simulink model "HW6SimulinkPID"  (R2017b)
settings: Solver=VariableStepAuto  StartTime=0.0  StopTime=TSim  RelTol=1e-3
values from neighbouring files (symbols this model uses):
  g = in(4)    [Gravity.m]    (also in TrajectoryGeneration1.m = 9.814; TrajectoryGeneration2.m = 9.814)
  init_th = (pi/180)*[0;30;0]    [PidGainMatrices1.m]    (also in PidGainMatrices2.m = (pi/180)*[15;15;15])
  init_thd = zeros(3,1)    [PidGainMatrices1.m]    (also in PidGainMatrices2.m)
  Kii = diag([ki1 ki2 ki3])    [PidGainMatrices1.m]    (also in PidGainMatrices2.m)
  Kpp = diag([kpp1 kpp2 kpp3])    [PidGainMatrices1.m]    (also in PidGainMatrices2.m)
  Kvv = diag([kvv1 kvv2 kvv3])    [PidGainMatrices1.m]    (also in PidGainMatrices2.m)
settings Model: Creator=JRizk  LastModifiedBy=JRizk

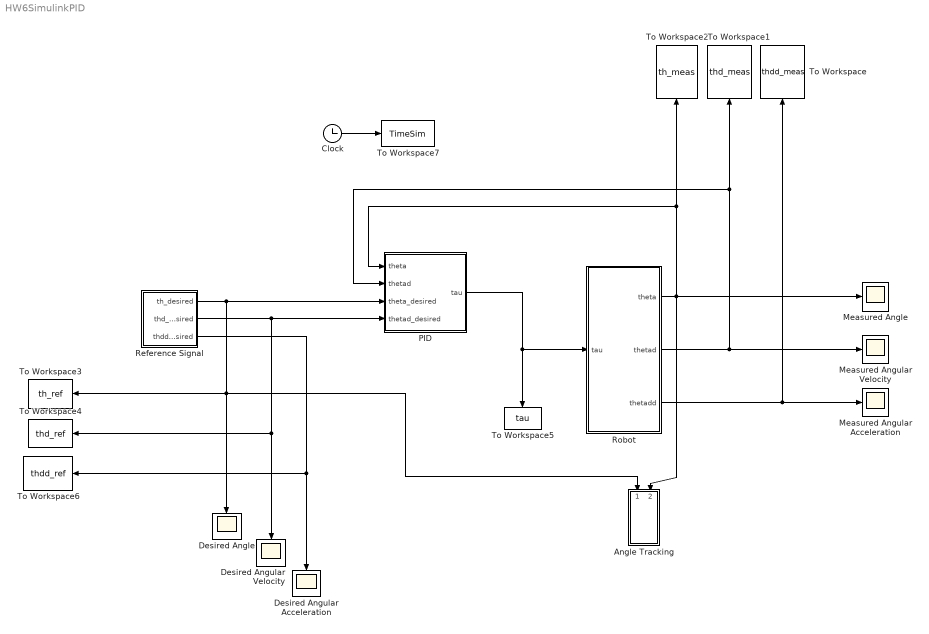
== system HW6SimulinkPID ==
  Angle Tracking : Subsystem
  Clock : Clock
  Desired Angle : Scope
  Desired Angular Acceleration : Scope
  Desired Angular Velocity : Scope
  Measured Angle : Scope
  Measured Angular Acceleration : Scope
  Measured Angular Velocity : Scope
  PID : Subsystem
  Reference Signal : Subsystem
  Robot : Subsystem
  To Workspace : ToWorkspace  VariableName=thdd_meas  SaveFormat=Timeseries  SampleTime=-1
  To Workspace1 : ToWorkspace  VariableName=thd_meas  SaveFormat=Timeseries  SampleTime=-1
  To Workspace2 : ToWorkspace  VariableName=th_meas  SaveFormat=Timeseries  SampleTime=-1
  To Workspace3 : ToWorkspace  VariableName=th_ref  SaveFormat=Timeseries  SampleTime=-1
  To Workspace4 : ToWorkspace  VariableName=thd_ref  SaveFormat=Timeseries  SampleTime=-1
  To Workspace5 : ToWorkspace  VariableName=tau  SaveFormat=Timeseries  SampleTime=-1
  To Workspace6 : ToWorkspace  VariableName=thdd_ref  SaveFormat=Timeseries  SampleTime=-1
  To Workspace7 : ToWorkspace  VariableName=TimeSim  SaveFormat=Timeseries  SampleTime=-1
  wires:
  Robot/2(thetad) -> Measured Angular Velocity/1, PID/2(thetad), To Workspace1/1
  Robot/1(theta) -> Angle Tracking/2(th_meas), Measured Angle/1, To Workspace2/1, PID/1(theta)
  Robot/3(thetadd) -> Measured Angular Acceleration/1, To Workspace/1
  Reference Signal/1(th_desired) -> Angle Tracking/1(th_desired), To Workspace3/1, Desired Angle/1, PID/3(theta_desired)
  Reference Signal/2(thd_desired) -> To Workspace4/1, Desired Angular Velocity/1, PID/4(thetad_desired)
  PID/1(tau) -> To Workspace5/1, Robot/1(tau)
  Reference Signal/3(thdd_desired) -> To Workspace6/1, Desired Angular Acceleration/1
  Clock/1 -> To Workspace7/1

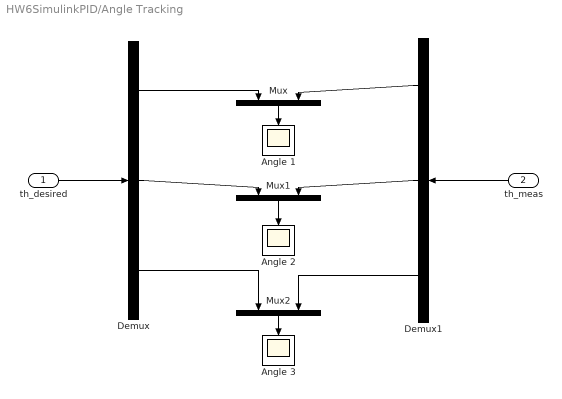
== system HW6SimulinkPID/Angle Tracking ==
  th_desired : Inport
  th_meas : Inport  Port=2
  Angle 1 : Scope
  Angle 2 : Scope
  Angle 3 : Scope
  Demux : Demux  Outputs=3
  Demux1 : Demux  Outputs=3
  Mux : Mux  Inputs=2
  Mux1 : Mux  Inputs=2
  Mux2 : Mux  Inputs=2
  wires:
  Mux/1 -> Angle 1/1
  Demux/2 -> Mux1/1
  th_meas/1 -> Demux1/1
  th_desired/1 -> Demux/1
  Demux/3 -> Mux2/1
  Demux1/1 -> Mux/2
  Mux2/1 -> Angle 3/1
  Demux1/3 -> Mux2/2
  Demux1/2 -> Mux1/2
  Demux/1 -> Mux/1
  Mux1/1 -> Angle 2/1

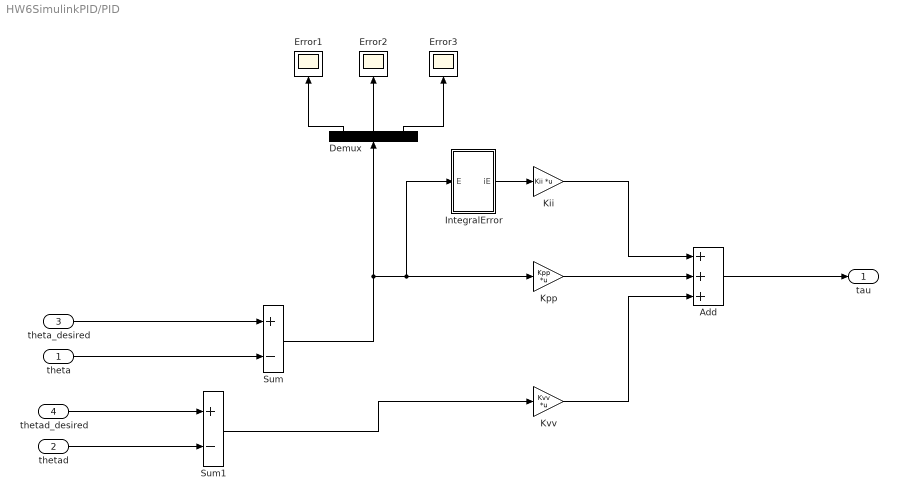
== system HW6SimulinkPID/PID ==
  theta : Inport
  thetad : Inport  Port=2
  theta_desired : Inport  Port=3
  thetad_desired : Inport  Port=4
  Add : Sum  Inputs=+++
  Demux : Demux  Outputs=3
  Error1 : Scope
  Error2 : Scope
  Error3 : Scope
  IntegralError : Subsystem
  Kii : Gain  Gain=Kii  Multiplication=Matrix(K*u)
  Kpp : Gain  Gain=Kpp  Multiplication=Matrix(K*u)
  Kvv : Gain  Gain=Kvv  Multiplication=Matrix(K*u)
  Sum : Sum  Inputs=+-
  Sum1 : Sum  Inputs=+-
  tau : Outport
  wires:
  theta_desired/1 -> Sum/1
  Demux/1 -> Error1/1
  Kpp/1 -> Add/2
  theta/1 -> Sum/2
  thetad/1 -> Sum1/2
  Sum/1 -> Demux/1, IntegralError/1(E), Kpp/1
  Kii/1 -> Add/1
  Kvv/1 -> Add/3
  Add/1 -> tau/1
  Sum1/1 -> Kvv/1
  thetad_desired/1 -> Sum1/1
  IntegralError/1(iE) -> Kii/1
  Demux/3 -> Error3/1
  Demux/2 -> Error2/1

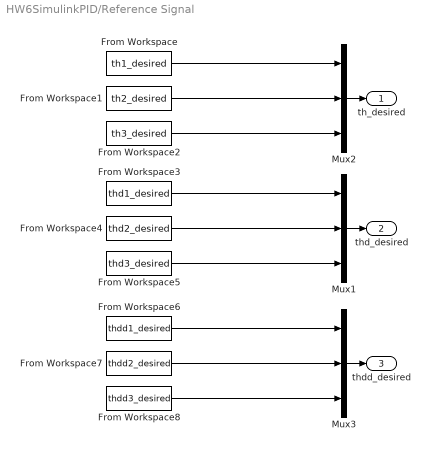
== system HW6SimulinkPID/Reference Signal ==
  From Workspace : FromWorkspace  VariableName=th1_desired
  From Workspace1 : FromWorkspace  VariableName=th2_desired
  From Workspace2 : FromWorkspace  VariableName=th3_desired
  From Workspace3 : FromWorkspace  VariableName=thd1_desired
  From Workspace4 : FromWorkspace  VariableName=thd2_desired
  From Workspace5 : FromWorkspace  VariableName=thd3_desired
  From Workspace6 : FromWorkspace  VariableName=thdd1_desired
  From Workspace7 : FromWorkspace  VariableName=thdd2_desired
  From Workspace8 : FromWorkspace  VariableName=thdd3_desired
  Mux1 : Mux  Inputs=3
  Mux2 : Mux  Inputs=3
  Mux3 : Mux  Inputs=3
  th_desired : Outport
  thd_desired : Outport  Port=2
  thdd_desired : Outport  Port=3
  wires:
  From Workspace3/1 -> Mux1/1
  From Workspace6/1 -> Mux3/1
  From Workspace4/1 -> Mux1/2
  From Workspace7/1 -> Mux3/2
  From Workspace/1 -> Mux2/1
  From Workspace1/1 -> Mux2/2
  From Workspace2/1 -> Mux2/3
  From Workspace8/1 -> Mux3/3
  From Workspace5/1 -> Mux1/3
  Mux2/1 -> th_desired/1
  Mux3/1 -> thdd_desired/1
  Mux1/1 -> thd_desired/1

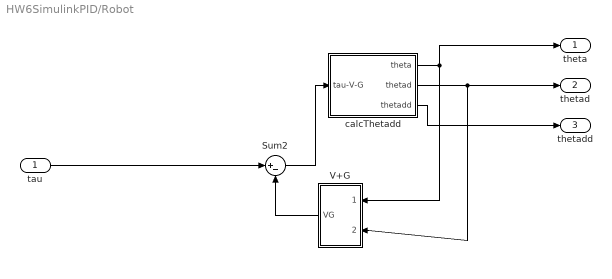
== system HW6SimulinkPID/Robot ==
  tau : Inport
  Sum2 : Sum  Inputs=|+-
  V+G : Subsystem
  calcThetadd : Subsystem
  theta : Outport
  thetad : Outport  Port=2
  thetadd : Outport  Port=3
  wires:
  calcThetadd/1(theta) -> V+G/1(theta), theta/1
  calcThetadd/2(thetad) -> V+G/2(thetad), thetad/1
  Sum2/1 -> calcThetadd/1(tau-V-G)
  calcThetadd/3(thetadd) -> thetadd/1
  tau/1 -> Sum2/1
  V+G/1(VG) -> Sum2/2

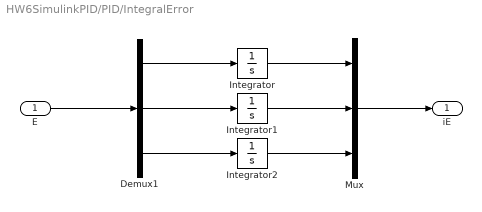
== system HW6SimulinkPID/PID/IntegralError ==
  E : Inport
  Demux1 : Demux  Outputs=3
  Integrator : Integrator
  Integrator1 : Integrator
  Integrator2 : Integrator
  Mux : Mux  Inputs=3
  iE : Outport
  wires:
  Demux1/1 -> Integrator/1
  Integrator1/1 -> Mux/2
  Demux1/2 -> Integrator1/1
  Integrator/1 -> Mux/1
  E/1 -> Demux1/1
  Integrator2/1 -> Mux/3
  Mux/1 -> iE/1
  Demux1/3 -> Integrator2/1

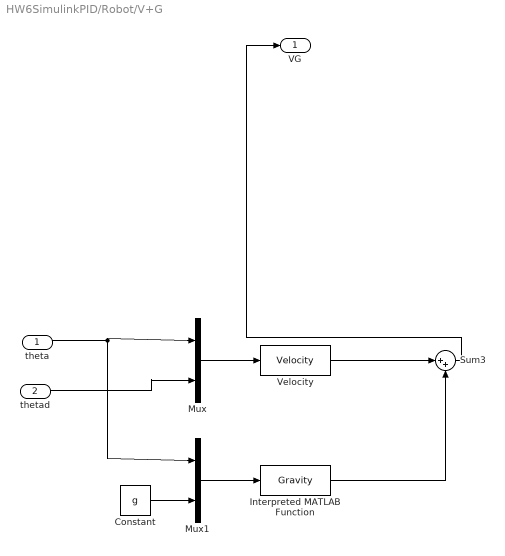
== system HW6SimulinkPID/Robot/V+G ==
  theta : Inport
  thetad : Inport  Port=2
  Constant : Constant  Value=g
  Interpreted MATLAB Function : MATLABFcn  MATLABFcn=Gravity  OutputDimensions=3
  Mux : Mux  Inputs=2
  Mux1 : Mux  Inputs=2
  Sum3 : Sum  Inputs=|++
  Velocity : MATLABFcn  MATLABFcn=Velocity  OutputDimensions=3
  VG : Outport
  wires:
  Interpreted MATLAB Function/1 -> Sum3/2
  Constant/1 -> Mux1/2
  Mux1/1 -> Interpreted MATLAB Function/1
  Velocity/1 -> Sum3/1
  Sum3/1 -> VG/1
  Mux/1 -> Velocity/1
  thetad/1 -> Mux/2
  theta/1 -> Mux1/1, Mux/1

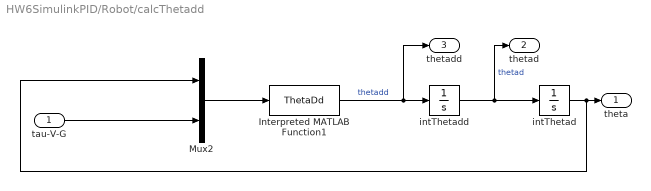
== system HW6SimulinkPID/Robot/calcThetadd ==
  tau-V-G : Inport
  Interpreted MATLAB Function1 : MATLABFcn  MATLABFcn=ThetaDd  OutputDimensions=3
  Mux2 : Mux  Inputs=2
  intThetad : Integrator  InitialCondition=init_th
  intThetadd : Integrator  InitialCondition=init_thd
  theta : Outport
  thetad : Outport  Port=2
  thetadd : Outport  Port=3
  wires:
  Interpreted MATLAB Function1/1 -> thetadd/1, intThetadd/1  "thetadd"
  tau-V-G/1 -> Mux2/2
  intThetad/1 -> Mux2/1, theta/1
  intThetadd/1 -> thetad/1, intThetad/1  "thetad"
  Mux2/1 -> Interpreted MATLAB Function1/1
